simulink model "MRAC_P1_sigmamod"  (R2019a)
settings: Solver=VariableStepAuto  StartTime=0.0  StopTime=1000  RelTol=1e-3
libraries: slctrlblks x3
settings Model: Creator=morga  LastModifiedBy=morga

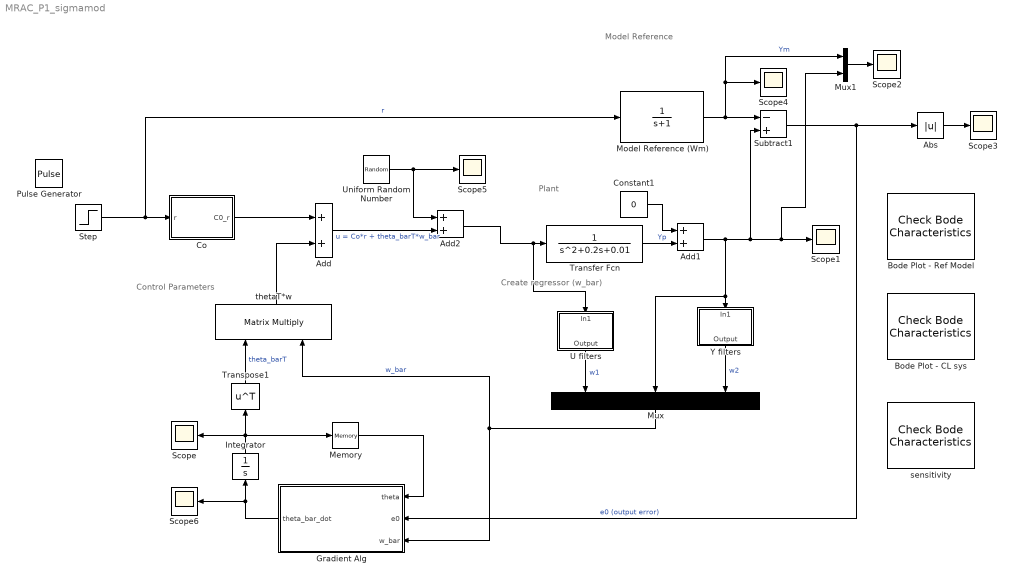
== system MRAC_P1_sigmamod ==
  note: Plant
  note: Model Reference
  note: Create regressor (w_bar)
  note: Control Parameters
  Abs : Abs
  Add : Sum
  Add1 : Sum
  Add2 : Sum
  Bode Plot - CL sys : slctrlblks/Model Verification/Check Bode  Characteristics  InstantiateOnLoad=on  SaveOperatingPoints=off  LinearizationIOs={'/Transfer Fcn', 1, 'out', 'off', '';'/Pulse Generator', 1, 'in', 'off', ''}  LinearizeAt=SnapshotTimes  SnapshotTimes=[0]  TriggerType=rising  SampleTime=auto  RateConversionMethod=zoh  PreWarpFreq=10  UseExactDelayModel=off  UseFullBlockNameLabels=off  UseBusSignalLabels=off  enabled=on  stopWhenAssertionFail=off  export=off  ViewDlgPos=[444 199 510 445.5]  OpenViewOnLoad=off  LaunchViewOnOpen=on  FrequencyUnits=rad/s  MagnitudeUnits=dB  PhaseUnits=deg  TimeUnits=seconds  EnableUpperBound=off  UpperBoundFrequencies=[]  UpperBoundMagnitudes=[]  EnableLowerBound=off  LowerBoundFrequencies=[]  LowerBoundMagnitudes=[]
      settings: SourceProductName=Simulink Control Design
  Bode Plot - Ref Model : slctrlblks/Model Verification/Check Bode  Characteristics  InstantiateOnLoad=on  SaveOperatingPoints=off  LinearizationIOs={'/Step', 1, 'in', 'off', '';'/Model Reference (Wm)', 1, 'out', 'on', ''}  LinearizeAt=SnapshotTimes  SnapshotTimes=[0]  TriggerType=rising  SampleTime=auto  RateConversionMethod=zoh  PreWarpFreq=10  UseExactDelayModel=off  UseFullBlockNameLabels=off  UseBusSignalLabels=off  enabled=on  stopWhenAssertionFail=off  export=off  ViewDlgPos=[2993 91 510 390]  OpenViewOnLoad=off  LaunchViewOnOpen=on  FrequencyUnits=rad/s  MagnitudeUnits=dB  PhaseUnits=deg  TimeUnits=seconds  EnableUpperBound=off  UpperBoundFrequencies=[]  UpperBoundMagnitudes=[]  EnableLowerBound=off  LowerBoundFrequencies=[]  LowerBoundMagnitudes=[]
      settings: SourceProductName=Simulink Control Design
  Co : MATLAB Function  TreatAsAtomicUnit=on
  Constant1 : Constant  Value=0
  Gradient Alg : MATLAB Function  TreatAsAtomicUnit=on
  Integrator : Integrator
  Memory : Memory
  Model Reference (Wm) : TransferFcn  Denominator=[1 1]
  Mux : Mux  Inputs=3
      settings: DisplayOption=signals
  Mux1 : Mux  Inputs=2
  Pulse Generator : DiscretePulseGenerator  PulseType=Time based  Period=1000  PulseWidth=25
  Scope{,1..6} (7 alike) : Scope
  Step : Step  Time=0  SampleTime=0
  Subtract1 : Sum  Inputs=-+
  Transfer Fcn : TransferFcn  Denominator=[1 0.2 0.01]
  Transpose1 : Math  Operator=transpose  SaturateOnIntegerOverflow=on
  U filters : Subsystem
  Uniform Random Number : UniformRandomNumber  Minimum=-0.1  Maximum=0.1  SampleTime=0.1
  Y filters : Subsystem
  sensitivity : slctrlblks/Model Verification/Check Bode  Characteristics  InstantiateOnLoad=on  SaveOperatingPoints=off  LinearizationIOs={'/Constant1', 1, 'in', 'off', '';'/Add1', 1, 'out', 'off', ''}  LinearizeAt=SnapshotTimes  SnapshotTimes=[0]  TriggerType=rising  SampleTime=auto  RateConversionMethod=zoh  PreWarpFreq=10  UseExactDelayModel=off  UseFullBlockNameLabels=off  UseBusSignalLabels=off  enabled=on  stopWhenAssertionFail=off  export=off  ViewDlgPos=[100 200 510 390]  OpenViewOnLoad=off  LaunchViewOnOpen=on  FrequencyUnits=rad/s  MagnitudeUnits=dB  PhaseUnits=deg  TimeUnits=seconds  EnableUpperBound=off  UpperBoundFrequencies=[]  UpperBoundMagnitudes=[]  EnableLowerBound=off  LowerBoundFrequencies=[]  LowerBoundMagnitudes=[]
      settings: SourceProductName=Simulink Control Design
  thetaT*w : Product  Multiplication=Matrix(*)
  wires:
  Step/1 -> Model Reference (Wm)/1, Co/1(r)  "r"
  Model Reference (Wm)/1 -> Mux1/1, Scope4/1, Subtract1/1  "Ym"
  U filters/1(Output) -> Mux/1  "w1"
  Co/1(C0_r) -> Add/1
  Y filters/1(Output) -> Mux/3  "w2"
  Mux/1 -> Gradient Alg/3(w_bar), thetaT*w/2  "w_bar"
  Transpose1/1 -> thetaT*w/1  "theta_barT"
  thetaT*w/1 -> Add/2
  Gradient Alg/1(theta_bar_dot) -> Integrator/1, Scope6/1
  Integrator/1 -> Transpose1/1, Memory/1, Scope/1
  Subtract1/1 -> Abs/1, Gradient Alg/2(e0)  "e0 (output error)"
  Mux1/1 -> Scope2/1
  Abs/1 -> Scope3/1
  Transfer Fcn/1 -> Add1/2  "Yp"
  Constant1/1 -> Add1/1
  Add1/1 -> Subtract1/2, Mux1/2, Scope1/1, Mux/2, Y filters/1(In1)
  Uniform Random Number/1 -> Add2/1, Scope5/1
  Add2/1 -> U filters/1(In1), Transfer Fcn/1
  Add/1 -> Add2/2  "u = Co*r + theta_barT*w_bar"
  Memory/1 -> Gradient Alg/1(theta)

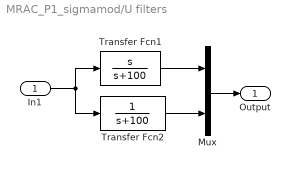
== system MRAC_P1_sigmamod/U filters ==
  In1 : Inport
  Mux : Mux  Inputs=2
  Transfer Fcn1 : TransferFcn  Numerator=[1 0]  Denominator=[1 100]
  Transfer Fcn2 : TransferFcn  Denominator=[1 100]
  Output : Outport
  wires:
  In1/1 -> Transfer Fcn1/1, Transfer Fcn2/1
  Transfer Fcn1/1 -> Mux/1
  Transfer Fcn2/1 -> Mux/2
  Mux/1 -> Output/1

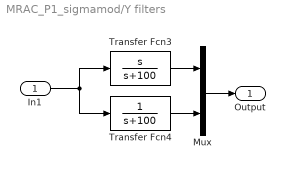
== system MRAC_P1_sigmamod/Y filters ==
  In1 : Inport
  Mux : Mux  Inputs=2
  Transfer Fcn3 : TransferFcn  Numerator=[1 0]  Denominator=[1 100]
  Transfer Fcn4 : TransferFcn  Denominator=[1 100]
  Output : Outport
  wires:
  In1/1 -> Transfer Fcn3/1, Transfer Fcn4/1
  Mux/1 -> Output/1
  Transfer Fcn3/1 -> Mux/1
  Transfer Fcn4/1 -> Mux/2

== matlab function MRAC_P1_sigmamod/Gradient Alg ==
  data: theta input; e0 input; theta_bar_dot output; w_bar input
function theta_bar_dot = fcn(theta, e0, w_bar)
g = 0.1; %adaptive gain
sigma = 0.001;
% theta_bar is vector of controller parameters of the form of [c', d0, d']
theta_bar_dot = -g * e0 * w_bar - sigma*theta;

== matlab function MRAC_P1_sigmamod/Co ==
  data: r input; C0_r output
function C0_r = fcn(r)
kp = 1;
km = 1; 
C0_star = km / kp;
C0_r = C0_star * r;
